simulink model "evtol_vehicle"  (R2024a)
settings: Solver=ode4  StartTime=0.0  StopTime=inf  FixedStep=0.01  RelTol=1e-3
values from neighbouring files (symbols this model uses):
  init_ned_m = waypoints(1:3,init_wypt_num)    [export_evtol_vehicle_fmu.m]
  init_rpy_rad = [0; waypoints(5,init_wypt_num); waypoints(4,init_wypt_num)] *pi/180    [export_evtol_vehicle_fmu.m]
  init_wypt_num = 1    [export_evtol_vehicle_fmu.m]
  max_hover_speed_mps = 15    [export_evtol_vehicle_fmu.m]
  num_waypoints = length(waypoints)    [export_evtol_vehicle_fmu.m]
  vdown_slew_rate_mps = 7.5    [export_evtol_vehicle_fmu.m]
  vx_slew_rate_mps = 7.5    [export_evtol_vehicle_fmu.m]
  vy_slew_rate_mps = 7.5    [export_evtol_vehicle_fmu.m]
  waypoints = [0 0 0 0 0 0 0 0 0 0 0 0 ... (900 elements, 9x100)]    [waypoints_empty.mat]
libraries: simulink x3, aerolibtransform2 x1
settings Model: Creator=cma  LastModifiedBy=Leo.Wong
settings OptimizationCC: ReuseModelBlockBuffer=off
settings RTWCC: GPUComputeCapability=3.5

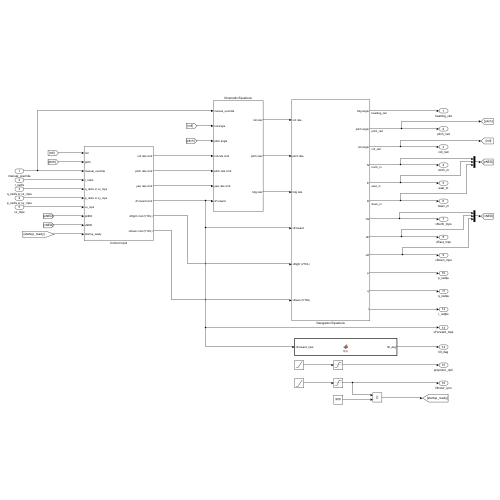
[thumbnail: Simulink's stored preview of the top-level diagram]
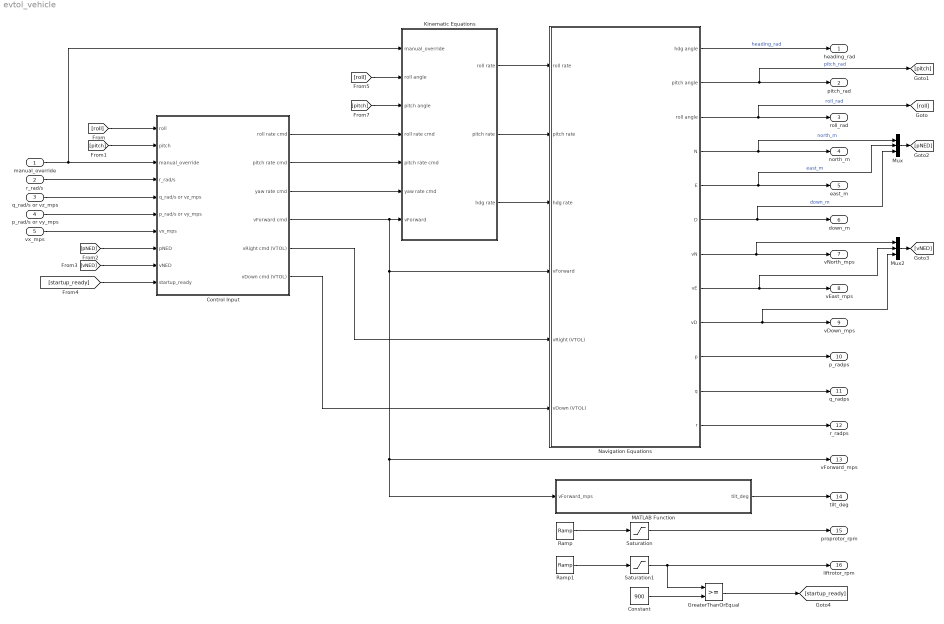
== system evtol_vehicle ==
  manual_override : Inport
  r_rad/s : Inport  Port=2
  q_rad/s or vz_mps : Inport  Port=3
  p_rad/s or vy_mps : Inport  Port=4
  vx_mps : Inport  Port=5
  Constant : Constant  Value=900
  Control Input : Subsystem  mask{wp_nedhgv=waypoints, num_wp=num_waypoints, initNED=init_ned_m, max_hover_speed=max_hover_speed_mps, vx_slew_rate=vx_slew_rate_mps, vy_slew_rate=vy_slew_rate_mps, vD_slew_rate=vdown_slew_rate_mps}
      mask prompts: wp_nedhgv "Waypoints"; num_wp "Number of Waypoints"; initNED "Initial NED (m)"; max_hover_speed "Max Hover Speed (mps)"; vx_slew_rate "Vx Slew Rate (mps)"; vy_slew_rate "Vy Slew Rate (mps)"; vD_slew_rate "VDown Slew Rate (mps)"
  GreaterThanOrEqual : RelationalOperator  OutDataTypeStr=boolean  RndMeth=Simplest  InputSameDT=off
  Kinematic Equations : Subsystem
  MATLAB Function : MATLAB Function  TreatAsAtomicUnit=on
  Mux : Mux  Inputs=3
  Mux2 : Mux  Inputs=3
  Navigation Equations : Subsystem  mask{initNED=init_ned_m, initRPY=init_rpy_rad}
      mask prompts: initNED "Initial NED (m)"; initRPY "Initial RPY (rad)"
  Ramp : simulink/Sources/Ramp  slope=600/5  start=0  InitialOutput=0
  Ramp1 : simulink/Sources/Ramp  slope=900/5  start=0  InitialOutput=0
  Saturation : Saturate  UpperLimit=600  LowerLimit=0
  Saturation1 : Saturate  UpperLimit=900  LowerLimit=0
  heading_rad : Outport
  pitch_rad : Outport  Port=2
  roll_rad : Outport  Port=3
  north_m : Outport  Port=4
  east_m : Outport  Port=5
  down_m : Outport  Port=6
  vNorth_mps : Outport  Port=7
  vEast_mps : Outport  Port=8
  vDown_mps : Outport  Port=9
  p_radps : Outport  Port=10
  q_radps : Outport  Port=11
  r_radps : Outport  Port=12
  vForward_mps : Outport  Port=13
  tilt_deg : Outport  Port=14
  proprotor_rpm : Outport  Port=15
  liftrotor_rpm : Outport  Port=16
  wires:
  Control Input/1(roll rate cmd) -> Kinematic Equations/4(roll rate cmd)
  Control Input/2(pitch rate cmd) -> Kinematic Equations/5(pitch rate cmd)
  Control Input/3(yaw rate cmd) -> Kinematic Equations/6(yaw rate cmd)
  [roll] -> Control Input/1(roll)
  [pitch] -> Control Input/2(pitch)
  Control Input/4(vForward cmd) -> Navigation Equations/4(vForward), MATLAB Function/1(vForward_mps), vForward_mps/1, Kinematic Equations/7(vForward)
  Control Input/6(vDown cmd (VTOL)) -> Navigation Equations/6(vDown (VTOL))
  Kinematic Equations/2(pitch rate) -> Navigation Equations/2(pitch rate)
  Kinematic Equations/1(roll rate) -> Navigation Equations/1(roll rate)
  Kinematic Equations/3(hdg rate) -> Navigation Equations/3(hdg rate)
  [roll] -> Kinematic Equations/2(roll angle)
  [pitch] -> Kinematic Equations/3(pitch angle)
  Control Input/5(vRight cmd (VTOL)) -> Navigation Equations/5(vRight (VTOL))
  r_rad/s/1 -> Control Input/4(r_rad/s)
  q_rad/s or vz_mps/1 -> Control Input/5(q_rad/s or vz_mps)
  p_rad/s or vy_mps/1 -> Control Input/6(p_rad/s or vy_mps)
  vx_mps/1 -> Control Input/7(vx_mps)
  Navigation Equations/4(N) -> Mux/1, north_m/1  "north_m"
  Navigation Equations/5(E) -> Mux/2, east_m/1  "east_m"
  Navigation Equations/6(D) -> Mux/3, down_m/1  "down_m"
  Navigation Equations/7(vN) -> Mux2/1, vNorth_mps/1
  Navigation Equations/8(vE) -> Mux2/2, vEast_mps/1
  Navigation Equations/9(vD) -> vDown_mps/1, Mux2/3
  Navigation Equations/10(p) -> p_radps/1
  Navigation Equations/11(q) -> q_radps/1
  Navigation Equations/12(r) -> r_radps/1
  Navigation Equations/3(roll angle) -> [roll], roll_rad/1  "roll_rad"
  Navigation Equations/2(pitch angle) -> [pitch], pitch_rad/1  "pitch_rad"
  Navigation Equations/1(hdg angle) -> heading_rad/1  "heading_rad"
  Mux/1 -> [pNED]
  Mux2/1 -> [vNED]
  manual_override/1 -> Kinematic Equations/1(manual_override), Control Input/3(manual_override)
  MATLAB Function/1(tilt_deg) -> tilt_deg/1
  Ramp/1 -> Saturation/1
  Ramp1/1 -> Saturation1/1
  Saturation/1 -> proprotor_rpm/1
  Saturation1/1 -> GreaterThanOrEqual/1, liftrotor_rpm/1
  [pNED] -> Control Input/8(pNED)
  [vNED] -> Control Input/9(vNED)
  GreaterThanOrEqual/1 -> [startup_ready]
  Constant/1 -> GreaterThanOrEqual/2
  [startup_ready] -> Control Input/10(startup_ready)

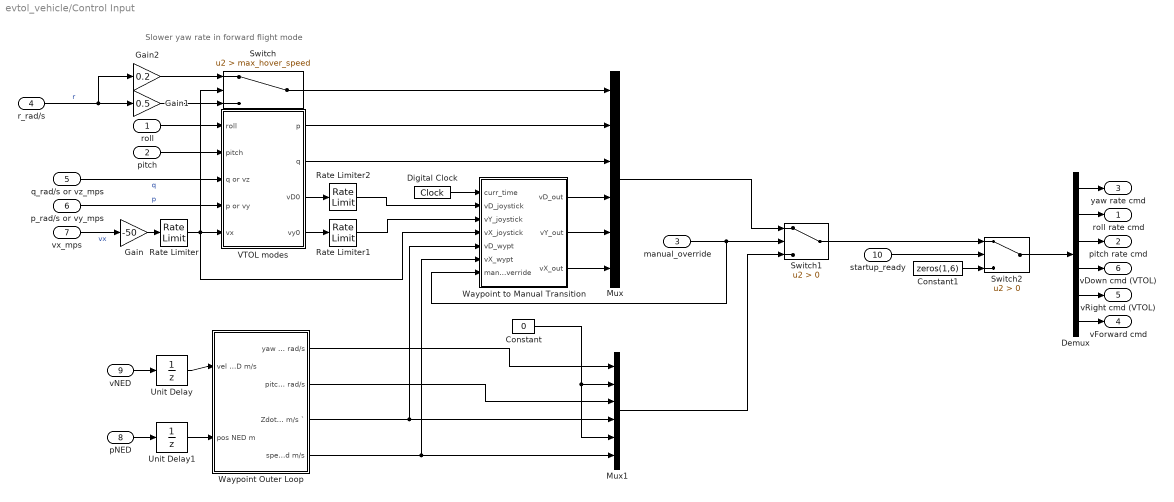
== system evtol_vehicle/Control Input ==
  note: Slower yaw rate in forward flight mode
  roll : Inport
  pitch : Inport  Port=2
  manual_override : Inport  Port=3
  r_rad/s : Inport  Port=4
  q_rad/s or vz_mps : Inport  Port=5
  p_rad/s or vy_mps : Inport  Port=6
  vx_mps : Inport  Port=7
  pNED : Inport  Port=8
  vNED : Inport  Port=9
  startup_ready : Inport  Port=10
  Constant : Constant  Value=0
  Constant1 : Constant  Value=zeros(1,6)
  Demux : Demux  Outputs=6
  Digital Clock : DigitalClock  SampleTime=0.01
  Gain : Gain  Gain=-50
  Gain1 : Gain  Gain=0.5
  Gain2 : Gain  Gain=0.2
  Mux : Mux  Inputs=6
  Mux1 : Mux  Inputs=6
  Rate Limiter : RateLimiter  RisingSlewLimit=vx_slew_rate  FallingSlewLimit=-vx_slew_rate  SampleTimeMode=inherited
  Rate Limiter1 : RateLimiter  RisingSlewLimit=vD_slew_rate  FallingSlewLimit=-vD_slew_rate  SampleTimeMode=inherited
  Rate Limiter2 : RateLimiter  RisingSlewLimit=vy_slew_rate  FallingSlewLimit=-vy_slew_rate  SampleTimeMode=inherited
  Switch : Switch  Criteria=u2 > Threshold  Threshold=max_hover_speed  SaturateOnIntegerOverflow=off  InputSameDT=off
  Switch1 : Switch  Criteria=u2 > Threshold  SaturateOnIntegerOverflow=off  InputSameDT=off
  Switch2 : Switch  Criteria=u2 > Threshold  SaturateOnIntegerOverflow=off  InputSameDT=off
  Unit Delay : UnitDelay  SampleTime=-1  HasFrameUpgradeWarning=on
  Unit Delay1 : UnitDelay  InitialCondition=initNED  SampleTime=-1  HasFrameUpgradeWarning=on
  VTOL modes : Subsystem
  Waypoint Outer Loop : Subsystem
  Waypoint to Manual Transition : MATLAB Function  TreatAsAtomicUnit=on  SystemSampleTime=0.01
  roll rate cmd : Outport
  pitch rate cmd : Outport  Port=2
  yaw rate cmd : Outport  Port=3
  vForward cmd : Outport  Port=4
  vRight cmd (VTOL) : Outport  Port=5
  vDown cmd (VTOL) : Outport  Port=6
  wires:
  Gain/1 -> Rate Limiter/1
  VTOL modes/3(vD0) -> Rate Limiter2/1
  r_rad/s/1 -> Gain2/1, Gain1/1  "r"
  p_rad/s or vy_mps/1 -> VTOL modes/4(p or vy)  "p"
  q_rad/s or vz_mps/1 -> VTOL modes/3(q or vz)  "q"
  vx_mps/1 -> Gain/1  "vx"
  roll/1 -> VTOL modes/1(roll)
  pitch/1 -> VTOL modes/2(pitch)
  VTOL modes/4(vy0) -> Rate Limiter1/1
  Gain2/1 -> Switch/1
  Gain1/1 -> Switch/3
  Rate Limiter/1 -> Waypoint to Manual Transition/4(vX_joystick), Switch/2, VTOL modes/5(vx)
  VTOL modes/2(q) -> Mux/3
  VTOL modes/1(p) -> Mux/2
  Mux/1 -> Switch1/1
  Demux/1 -> yaw rate cmd/1
  Demux/2 -> roll rate cmd/1
  Demux/3 -> pitch rate cmd/1
  Demux/4 -> vDown cmd (VTOL)/1
  Demux/5 -> vRight cmd (VTOL)/1
  Demux/6 -> vForward cmd/1
  Waypoint Outer Loop/4(speedCmd m/s) -> Waypoint to Manual Transition/6(vX_wypt), Mux1/6
  Waypoint Outer Loop/1(yaw rate rad/s) -> Mux1/1
  Waypoint Outer Loop/2(pitch rate rad/s) -> Mux1/3
  Waypoint Outer Loop/3(ZdotCmd m/s `) -> Waypoint to Manual Transition/5(vD_wypt), Mux1/4
  Mux1/1 -> Switch1/3
  Constant/1 -> Mux1/5, Mux1/2
  pNED/1 -> Unit Delay1/1
  manual_override/1 -> Waypoint to Manual Transition/7(manual_override), Switch1/2
  vNED/1 -> Unit Delay/1
  Switch/1 -> Mux/1
  Unit Delay/1 -> Waypoint Outer Loop/1(vel NED m/s)
  Unit Delay1/1 -> Waypoint Outer Loop/2(pos NED m)
  Switch1/1 -> Switch2/1
  Switch2/1 -> Demux/1
  startup_ready/1 -> Switch2/2
  Constant1/1 -> Switch2/3
  Digital Clock/1 -> Waypoint to Manual Transition/1(curr_time)
  Waypoint to Manual Transition/1(vD_out) -> Mux/4
  Waypoint to Manual Transition/2(vY_out) -> Mux/5
  Waypoint to Manual Transition/3(vX_out) -> Mux/6
  Rate Limiter2/1 -> Waypoint to Manual Transition/2(vD_joystick)
  Rate Limiter1/1 -> Waypoint to Manual Transition/3(vY_joystick)

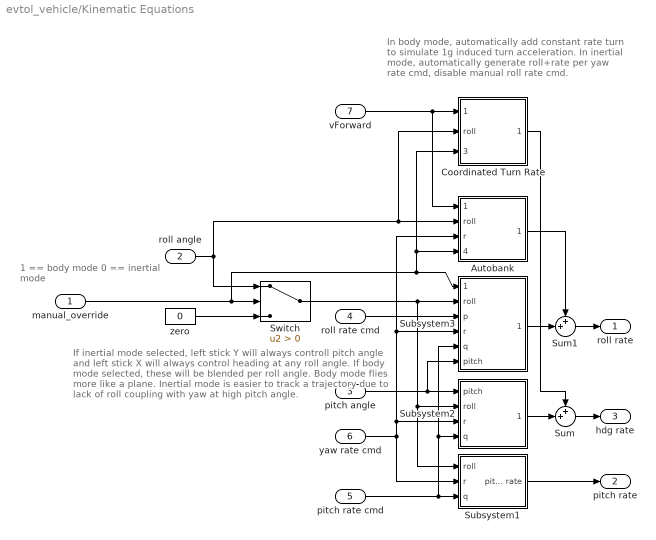
== system evtol_vehicle/Kinematic Equations ==
  note: If inertial mode selected, left stick Y will always controll pitch angle
      | and left stick X will always control heading at any roll angle.
      | If body mode selected, these will be blended per roll angle.
      | Body mode flies more like a plane.
      | Inertial mode is easier to track a trajectory due to lack
      | of roll coupling with yaw at high pitch angle.
  note: In body mode, automatically add constant rate
      | turn to simulate 1g induced turn acceleration.
      | In inertial mode, automatically generate roll+rate
      | per yaw rate cmd, disable manual roll rate cmd.
  note: 1 == body mode
      | 0 == inertial mode
  manual_override : Inport
  roll angle : Inport  Port=2
  pitch angle : Inport  Port=3
  roll rate cmd : Inport  Port=4
  pitch rate cmd : Inport  Port=5
  yaw rate cmd : Inport  Port=6
  vForward : Inport  Port=7
  Autobank : Subsystem
  Coordinated Turn Rate : Subsystem
  Subsystem1 : Subsystem
  Subsystem2 : Subsystem
  Subsystem3 : Subsystem
  Sum : Sum  Inputs=++|
  Sum1 : Sum  Inputs=++|
  Switch : Switch  Criteria=u2 > Threshold  SaturateOnIntegerOverflow=off  InputSameDT=off
  zero : Constant  Value=0
  roll rate : Outport
  pitch rate : Outport  Port=2
  hdg rate : Outport  Port=3
  wires:
  Subsystem1/1(pitch rate) -> pitch rate/1
  pitch rate cmd/1 -> Subsystem3/5(q), Subsystem2/4(q), Subsystem1/3(q)
  roll rate cmd/1 -> Subsystem3/3(p)
  yaw rate cmd/1 -> Subsystem1/2(r), Autobank/3(r), Subsystem3/4(r), Subsystem2/3(r)
  pitch angle/1 -> Subsystem3/6(pitch), Subsystem2/1(pitch)
  Switch/1 -> Subsystem1/1(roll), Subsystem2/2(roll), Subsystem3/2(roll)
  manual_override/1 -> Autobank/4(body mode), Coordinated Turn Rate/3(body mode), Subsystem3/1(body mode), Switch/2
  roll angle/1 -> Coordinated Turn Rate/2(roll), Autobank/2(roll), Switch/1
  zero/1 -> Switch/3
  Subsystem2/1(hdg rate) -> Sum/2
  Sum/1 -> hdg rate/1
  Coordinated Turn Rate/1(hdg rate) -> Sum/1
  vForward/1 -> Autobank/1(vForward), Coordinated Turn Rate/1(vForward)
  Sum1/1 -> roll rate/1
  Subsystem3/1(roll rate) -> Sum1/2
  Autobank/1(roll rate) -> Sum1/1

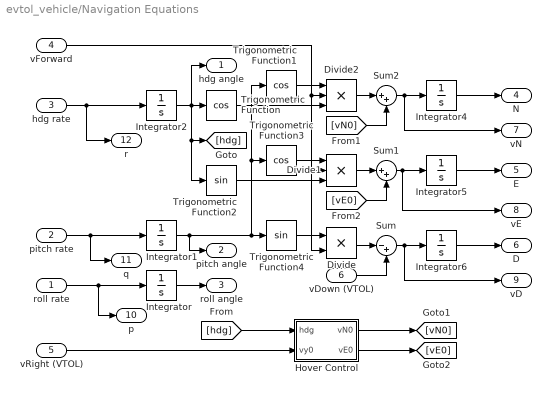
== system evtol_vehicle/Navigation Equations ==
  roll rate : Inport
  pitch rate : Inport  Port=2
  hdg rate : Inport  Port=3
  vForward : Inport  Port=4
  vRight (VTOL) : Inport  Port=5
  vDown (VTOL) : Inport  Port=6
  Divide : Product  Inputs=**
  Divide1 : Product  Inputs=***
  Divide2 : Product  Inputs=***
  Hover Control : Subsystem
  Integrator : Integrator  InitialCondition=initRPY(1)
  Integrator1 : Integrator  InitialCondition=initRPY(2)
  Integrator2 : Integrator  InitialCondition=initRPY(3)
  Integrator4 : Integrator  InitialCondition=initNED(1)
  Integrator5 : Integrator  InitialCondition=initNED(2)
  Integrator6 : Integrator  InitialCondition=initNED(3)
  Sum : Sum  Inputs=|-+
  Sum1 : Sum  Inputs=|++
  Sum2 : Sum  Inputs=|++
  Trigonometric Function : Trigonometry  Operator=cos
  Trigonometric Function1 : Trigonometry  Operator=cos
  Trigonometric Function2 : Trigonometry
  Trigonometric Function3 : Trigonometry  Operator=cos
  Trigonometric Function4 : Trigonometry
  hdg angle : Outport
  pitch angle : Outport  Port=2
  roll angle : Outport  Port=3
  N : Outport  Port=4
  E : Outport  Port=5
  D : Outport  Port=6
  vN : Outport  Port=7
  vE : Outport  Port=8
  vD : Outport  Port=9
  p : Outport  Port=10
  q : Outport  Port=11
  r : Outport  Port=12
  wires:
  Trigonometric Function3/1 -> Divide1/1
  Divide2/1 -> Sum2/1
  Trigonometric Function1/1 -> Divide2/1
  Sum/1 -> vD/1, Integrator6/1
  Divide/1 -> Sum/1
  Integrator1/1 -> pitch angle/1, Trigonometric Function1/1, Trigonometric Function3/1, Trigonometric Function4/1
  Divide1/1 -> Sum1/1
  Integrator2/1 -> hdg angle/1, [hdg], Trigonometric Function2/1, Trigonometric Function/1
  Trigonometric Function/1 -> Divide2/3
  Trigonometric Function4/1 -> Divide/1
  Sum2/1 -> vN/1, Integrator4/1
  Sum1/1 -> vE/1, Integrator5/1
  Trigonometric Function2/1 -> Divide1/3
  Integrator6/1 -> D/1
  vDown (VTOL)/1 -> Sum/2
  [vE0] -> Sum1/2
  [vN0] -> Sum2/2
  Integrator5/1 -> E/1
  Integrator4/1 -> N/1
  hdg rate/1 -> r/1, Integrator2/1
  roll rate/1 -> p/1, Integrator/1
  pitch rate/1 -> q/1, Integrator1/1
  Integrator/1 -> roll angle/1
  Hover Control/1(vN0) -> [vN0]
  Hover Control/2(vE0) -> [vE0]
  [hdg] -> Hover Control/1(hdg)
  vForward/1 -> Divide/2, Divide1/2, Divide2/2
  vRight (VTOL)/1 -> Hover Control/2(vy0)

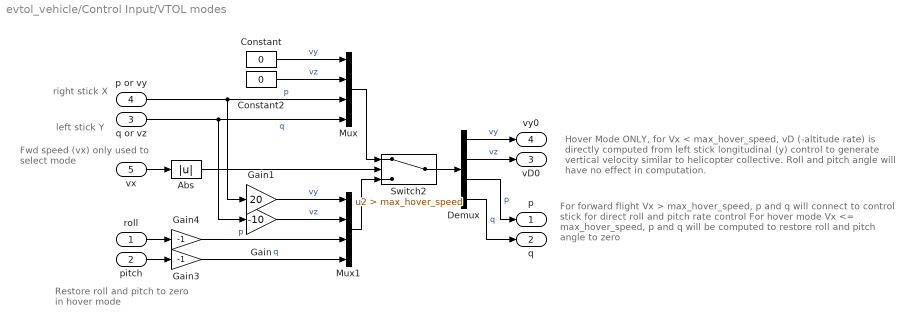
== system evtol_vehicle/Control Input/VTOL modes ==
  note: right stick X
  note: Fwd speed (vx) only
      | used to select mode
  note: Restore roll and pitch
      | to zero in hover mode
  note: Hover Mode ONLY, for Vx < max_hover_speed,
      | vD (-altitude rate) is directly computed from left stick longitudinal (y)
      | control to generate vertical velocity similar to helicopter collective.
      | Roll and pitch angle will have no effect in computation.
  note: For forward flight Vx > max_hover_speed, p and q will connect to
      | control stick for direct roll and pitch rate control
      |
      | For hover mode Vx <= max_hover_speed, p and q will be computed
      | to restore roll and pitch angle to zero
  note: left stick Y
  roll : Inport
  pitch : Inport  Port=2
  q or vz : Inport  Port=3
  p or vy : Inport  Port=4
  vx : Inport  Port=5
  Abs : Abs  SaturateOnIntegerOverflow=off
  Constant : Constant  Value=0
  Constant2 : Constant  Value=0
  Demux : Demux
  Gain : Gain  Gain=-10
  Gain1 : Gain  Gain=20
  Gain3 : Gain  Gain=-1
  Gain4 : Gain  Gain=-1
  Mux : Mux
  Mux1 : Mux
  Switch2 : Switch  Criteria=u2 > Threshold  Threshold=max_hover_speed  SaturateOnIntegerOverflow=off  InputSameDT=off
  p : Outport
  q : Outport  Port=2
  vD0 : Outport  Port=3
  vy0 : Outport  Port=4
  wires:
  Abs/1 -> Switch2/2
  Constant/1 -> Mux/1  "vy"
  vx/1 -> Abs/1
  p or vy/1 -> Gain1/1, Mux/3  "p"
  q or vz/1 -> Gain/1, Mux/4  "q"
  pitch/1 -> Gain3/1
  roll/1 -> Gain4/1
  Switch2/1 -> Demux/1
  Mux/1 -> Switch2/1
  Mux1/1 -> Switch2/3
  Gain1/1 -> Mux1/1  "vy"
  Constant2/1 -> Mux/2  "vz"
  Gain/1 -> Mux1/2  "vz"
  Gain3/1 -> Mux1/4  "q"
  Gain4/1 -> Mux1/3  "p"
  Demux/4 -> q/1  "q"
  Demux/3 -> p/1  "p"
  Demux/2 -> vD0/1  "vz"
  Demux/1 -> vy0/1  "vy"

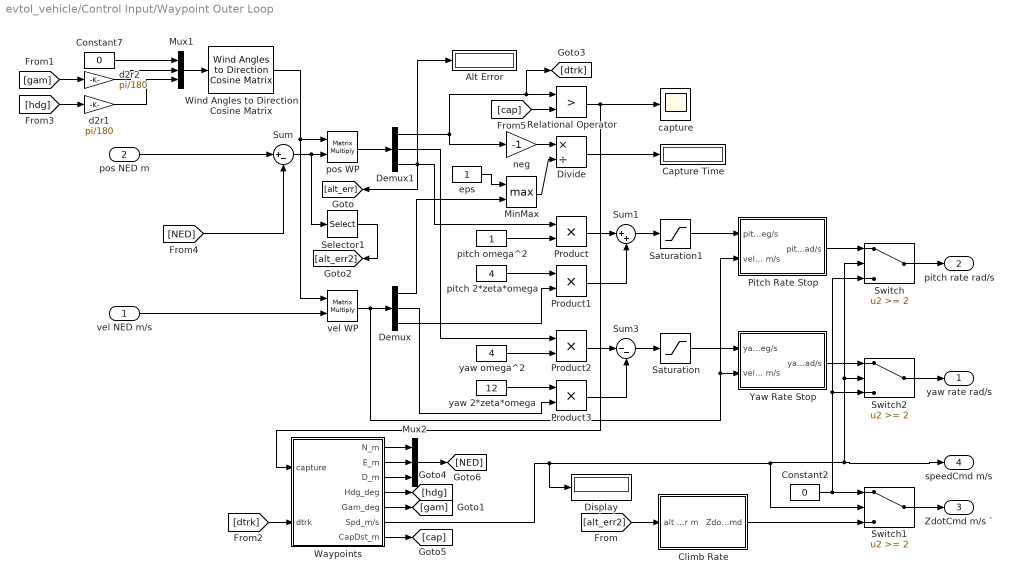
== system evtol_vehicle/Control Input/Waypoint Outer Loop ==
  vel NED m/s : Inport
  pos NED m : Inport  Port=2
  Alt Error : Display
  Capture Time : Display
  Climb Rate : Subsystem
  Constant2 : Constant  Value=0
  Constant7 : Constant  Value=0
  Demux : Demux  Outputs=3
  Demux1 : Demux  Outputs=3
  Display : Display
  Divide : Product  Inputs=*/
  MinMax : MinMax  Function=max  Inputs=2
  Mux1 : Mux  Inputs=3
  Mux2 : Mux  Inputs=3
  Pitch Rate Stop : Subsystem
  Product{,1..3} (4 alike) : Product
  Relational Operator : RelationalOperator  Operator=>  OutDataTypeStr=boolean  RndMeth=Simplest  InputSameDT=off
  Saturation : Saturate  UpperLimit=15  LowerLimit=-15
  Saturation1 : Saturate  UpperLimit=10  LowerLimit=-10
  Selector1 : Selector  InputPortWidth=3  IndexOptions=Index vector (dialog)  Indices=[3]  OutputSizes=1
  Sum : Sum  Inputs=|+-
  Sum1 : Sum  Inputs=|++
  Sum3 : Sum  Inputs=|--
  Switch : Switch  Threshold=2  SaturateOnIntegerOverflow=off  InputSameDT=off
  Switch1 : Switch  Threshold=2  SaturateOnIntegerOverflow=off  InputSameDT=off
  Switch2 : Switch  Threshold=2  SaturateOnIntegerOverflow=off  InputSameDT=off
  Waypoints : Subsystem
  Wind Angles to Direction Cosine Matrix : aerolibtransform2/Wind Angles to  Direction Cosine Matrix
  Yaw Rate Stop : Subsystem
  capture : Scope
  d2r1 : Gain  Gain=pi/180
  d2r2 : Gain  Gain=pi/180
  eps : Constant
  neg : Gain  Gain=-1
  pitch 2*zeta*omega : Constant  Value=4
  pitch omega^2 : Constant
  pos WP : Product  Multiplication=Matrix(*)
  vel WP : Product  Multiplication=Matrix(*)
  yaw 2*zeta*omega : Constant  Value=12
  yaw omega^2 : Constant  Value=4
  yaw rate rad/s : Outport
  pitch rate rad/s : Outport  Port=2
  ZdotCmd m/s ` : Outport  Port=3
  speedCmd m/s : Outport  Port=4
  wires:
  Sum/1 -> Selector1/1, pos WP/2
  Mux1/1 -> Wind Angles to Direction Cosine Matrix/1
  Constant7/1 -> Mux1/1
  Wind Angles to Direction Cosine Matrix/1 -> vel WP/1, pos WP/1
  pos WP/1 -> Demux1/1
  vel NED m/s/1 -> vel WP/2
  [NED] -> Sum/2
  pos NED m/1 -> Sum/1
  Demux1/1 -> neg/1, [dtrk], Relational Operator/1
  [cap] -> Relational Operator/2
  Relational Operator/1 -> capture/1, Waypoints/1(capture)
  Sum1/1 -> Saturation1/1
  Product/1 -> Sum1/1
  Product1/1 -> Sum1/2
  pitch omega^2/1 -> Product/2
  pitch 2*zeta*omega/1 -> Product1/1
  Demux1/3 -> [alt_err], Alt Error/1, Product/1
  yaw 2*zeta*omega/1 -> Product3/1
  yaw omega^2/1 -> Product2/2
  Product3/1 -> Sum3/2
  Product2/1 -> Sum3/1
  Sum3/1 -> Saturation/1
  Demux1/2 -> Product2/1
  neg/1 -> Divide/1
  Divide/1 -> Capture Time/1
  Demux/3 -> Product1/2
  Demux/2 -> Product3/2
  MinMax/1 -> Divide/2
  eps/1 -> MinMax/1
  Demux/1 -> MinMax/2
  vel WP/1 -> Pitch Rate Stop/2(vel WP m/s), Yaw Rate Stop/2(vel WP m/s), Demux/1
  Saturation1/1 -> Pitch Rate Stop/1(pitch rate Cmd deg/s)
  Waypoints/6(Spd_m/s) -> Display/1, Switch/2, Switch2/2, speedCmd m/s/1, Switch1/2
  d2r1/1 -> Mux1/3
  d2r2/1 -> Mux1/2
  Pitch Rate Stop/1(pitch rate rad/s) -> Switch/1
  Switch/1 -> pitch rate rad/s/1
  Constant2/1 -> Switch1/1, Switch2/3, Switch/3
  [alt_err2] -> Climb Rate/1(alt error m)
  Switch1/1 -> ZdotCmd m/s `/1
  Climb Rate/1(ZdotCmd) -> Switch1/3
  Saturation/1 -> Yaw Rate Stop/1(yaw rate Cmd deg/s)
  Selector1/1 -> [alt_err2]
  [dtrk] -> Waypoints/2(dtrk)
  Waypoints/5(Gam_deg) -> [gam]
  Waypoints/4(Hdg_deg) -> [hdg]
  Waypoints/7(CapDst_m) -> [cap]
  [hdg] -> d2r1/1
  [gam] -> d2r2/1
  Waypoints/1(N_m) -> Mux2/1
  Waypoints/2(E_m) -> Mux2/2
  Waypoints/3(D_m) -> Mux2/3
  Mux2/1 -> [NED]
  Yaw Rate Stop/1(yaw rate rad/s) -> Switch2/1
  Switch2/1 -> yaw rate rad/s/1

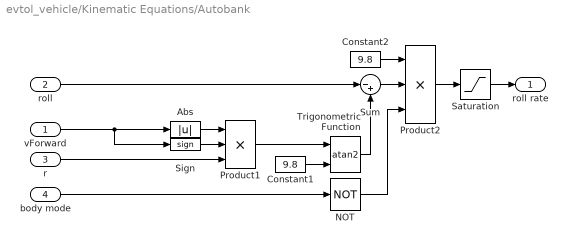
== system evtol_vehicle/Kinematic Equations/Autobank ==
  vForward : Inport
  roll : Inport  Port=2
  r : Inport  Port=3
  body mode : Inport  Port=4
  Abs : Abs  SaturateOnIntegerOverflow=off
  Constant1 : Constant  Value=9.8
  Constant2 : Constant  Value=9.8
  NOT : Logic  Operator=NOT  IconShape=distinctive  AllPortsSameDT=off  OutDataTypeStr=boolean
  Product1 : Product  Inputs=3
  Product2 : Product  Inputs=3
  Saturation : Saturate  UpperLimit=45*pi/180  LowerLimit=-45*pi/180
  Sign : Signum
  Sum : Sum  Inputs=|-+
  Trigonometric Function : Trigonometry  Operator=atan2
  roll rate : Outport
  wires:
  Abs/1 -> Product1/1
  Product1/1 -> Trigonometric Function/1
  vForward/1 -> Sign/1, Abs/1
  Constant1/1 -> Trigonometric Function/2
  roll/1 -> Sum/1
  Trigonometric Function/1 -> Sum/2
  Product2/1 -> Saturation/1
  Sum/1 -> Product2/2
  Constant2/1 -> Product2/1
  body mode/1 -> NOT/1
  NOT/1 -> Product2/3
  Sign/1 -> Product1/2
  r/1 -> Product1/3
  Saturation/1 -> roll rate/1

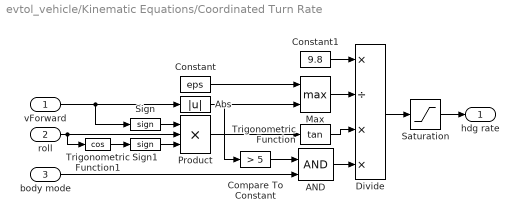
== system evtol_vehicle/Kinematic Equations/Coordinated Turn Rate ==
  vForward : Inport
  roll : Inport  Port=2
  body mode : Inport  Port=3
  AND : Logic  IconShape=distinctive  AllPortsSameDT=off  OutDataTypeStr=boolean
  Abs : Abs  SaturateOnIntegerOverflow=off
  Compare To Constant : simulink/Logic and Bit Operations/Compare To Constant  relop=>  const=5  OutDataTypeStr=boolean
  Constant : Constant  Value=eps
  Constant1 : Constant  Value=9.8
  Divide : Product  Inputs=*/**
  Max : MinMax  Function=max  Inputs=2
  Product : Product  Inputs=3
  Saturation : Saturate  UpperLimit=1  LowerLimit=-1
  Sign : Signum
  Sign1 : Signum
  Trigonometric Function : Trigonometry  Operator=tan
  Trigonometric Function1 : Trigonometry  Operator=cos
  hdg rate : Outport
  wires:
  Sign/1 -> Product/1
  Constant/1 -> Max/1
  Constant1/1 -> Divide/1
  vForward/1 -> Sign/1, Abs/1
  Product/1 -> Trigonometric Function/1
  Divide/1 -> Saturation/1
  Max/1 -> Divide/2
  Compare To Constant/1 -> AND/1
  AND/1 -> Divide/4
  Saturation/1 -> hdg rate/1
  Trigonometric Function/1 -> Divide/3
  Abs/1 -> Compare To Constant/1, Max/2
  body mode/1 -> AND/2
  roll/1 -> Product/2, Trigonometric Function1/1
  Sign1/1 -> Product/3
  Trigonometric Function1/1 -> Sign1/1

== system evtol_vehicle/Kinematic Equations/Subsystem1 ==
  roll : Inport
  r : Inport  Port=2
  q : Inport  Port=3
  Divide4 : Product  Inputs=**
  Divide6 : Product  Inputs=**
  Sum : Sum  Inputs=|+-
  Trigonometric Function7 : Trigonometry  Operator=cos
  Trigonometric Function8 : Trigonometry
  pitch rate : Outport
  wires:
  r/1 -> Divide6/2
  Trigonometric Function8/1 -> Divide6/1
  Divide6/1 -> Sum/2
  Trigonometric Function7/1 -> Divide4/2
  Divide4/1 -> Sum/1
  Sum/1 -> pitch rate/1
  roll/1 -> Trigonometric Function7/1, Trigonometric Function8/1
  q/1 -> Divide4/1

== system evtol_vehicle/Kinematic Equations/Subsystem2 ==
  pitch : Inport
  roll : Inport  Port=2
  r : Inport  Port=3
  q : Inport  Port=4
  Divide : Product  Inputs=*/
  Divide3 : Product  Inputs=**
  Divide5 : Product  Inputs=**
  Sum1 : Sum  Inputs=++|
  Trigonometric Function1 : Trigonometry  Operator=cos
  Trigonometric Function5 : Trigonometry  Operator=cos
  Trigonometric Function6 : Trigonometry
  hdg rate : Outport
  wires:
  roll/1 -> Trigonometric Function5/1, Trigonometric Function6/1
  Trigonometric Function5/1 -> Divide3/2
  r/1 -> Divide3/1
  Trigonometric Function6/1 -> Divide5/1
  Divide5/1 -> Sum1/2
  Divide3/1 -> Sum1/1
  q/1 -> Divide5/2
  pitch/1 -> Trigonometric Function1/1
  Sum1/1 -> Divide/1
  Divide/1 -> hdg rate/1
  Trigonometric Function1/1 -> Divide/2

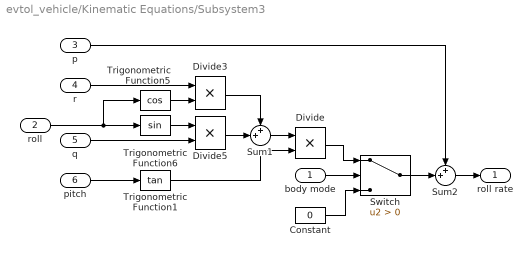
== system evtol_vehicle/Kinematic Equations/Subsystem3 ==
  body mode : Inport
  roll : Inport  Port=2
  p : Inport  Port=3
  r : Inport  Port=4
  q : Inport  Port=5
  pitch : Inport  Port=6
  Constant : Constant  Value=0
  Divide : Product  Inputs=**
  Divide3 : Product  Inputs=**
  Divide5 : Product  Inputs=**
  Sum1 : Sum  Inputs=++|
  Sum2 : Sum  Inputs=++|
  Switch : Switch  Criteria=u2 > Threshold  SaturateOnIntegerOverflow=off  InputSameDT=off
  Trigonometric Function1 : Trigonometry  Operator=tan
  Trigonometric Function5 : Trigonometry  Operator=cos
  Trigonometric Function6 : Trigonometry
  roll rate : Outport
  wires:
  Trigonometric Function1/1 -> Divide/2
  Sum1/1 -> Divide/1
  pitch/1 -> Trigonometric Function1/1
  q/1 -> Divide5/2
  Trigonometric Function6/1 -> Divide5/1
  r/1 -> Divide3/1
  Trigonometric Function5/1 -> Divide3/2
  roll/1 -> Trigonometric Function6/1, Trigonometric Function5/1
  Divide5/1 -> Sum1/2
  Divide3/1 -> Sum1/1
  Sum2/1 -> roll rate/1
  p/1 -> Sum2/1
  body mode/1 -> Switch/2
  Divide/1 -> Switch/1
  Switch/1 -> Sum2/2
  Constant/1 -> Switch/3

== system evtol_vehicle/Navigation Equations/Hover Control ==
  note: heading is used to distribute
      | lateral velocity vy to vN and vE
  note: Hover Mode ONLY, for Vx < max_hover_speed_mps,
      | vE and vN are directly computed from right stick lateral (x)
      | control to generate lateral translation velocity based on heading.
      | Roll and pitch angle will have no effect in compuation.
  hdg : Inport
  vy0 : Inport  Port=2
  Constant1 : Constant  Value=-1
  Product : Product  Inputs=3
  Product1 : Product
  Trigonometric Function : Trigonometry  Operator=cos
  Trigonometric Function1 : Trigonometry
  vN0 : Outport
  vE0 : Outport  Port=2
  wires:
  vy0/1 -> Product1/2, Product/2
  Product1/1 -> vE0/1
  Trigonometric Function1/1 -> Product/1
  Product/1 -> vN0/1
  hdg/1 -> Trigonometric Function1/1, Trigonometric Function/1
  Constant1/1 -> Product/3
  Trigonometric Function/1 -> Product1/1

== system evtol_vehicle/Control Input/Waypoint Outer Loop/Climb Rate ==
  alt error m : Inport
  Constant3 : Constant  Value=-1
  Product5 : Product
  Saturation2 : Saturate  UpperLimit=5  LowerLimit=-5
  ZdotCmd : Outport
  wires:
  Constant3/1 -> Product5/2
  Product5/1 -> Saturation2/1
  alt error m/1 -> Product5/1
  Saturation2/1 -> ZdotCmd/1

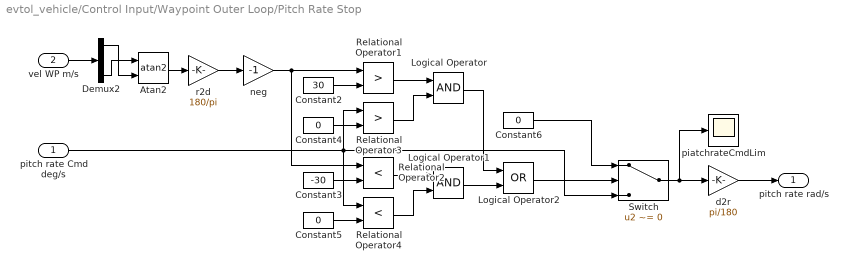
== system evtol_vehicle/Control Input/Waypoint Outer Loop/Pitch Rate Stop ==
  pitch rate Cmd deg/s : Inport
  vel WP m/s : Inport  Port=2
  Atan2 : Trigonometry  Operator=atan2
  Constant2 : Constant  Value=30
  Constant3 : Constant  Value=-30
  Constant4 : Constant  Value=0
  Constant5 : Constant  Value=0
  Constant6 : Constant  Value=0
  Demux2 : Demux  Outputs=3
  Logical Operator : Logic  AllPortsSameDT=off  OutDataTypeStr=boolean
  Logical Operator1 : Logic  AllPortsSameDT=off  OutDataTypeStr=boolean
  Logical Operator2 : Logic  Operator=OR  AllPortsSameDT=off  OutDataTypeStr=boolean
  Relational Operator1 : RelationalOperator  Operator=>  OutDataTypeStr=boolean  RndMeth=Simplest  InputSameDT=off
  Relational Operator2 : RelationalOperator  Operator=<  OutDataTypeStr=boolean  RndMeth=Simplest  InputSameDT=off
  Relational Operator3 : RelationalOperator  Operator=>  OutDataTypeStr=boolean  RndMeth=Simplest  InputSameDT=off
  Relational Operator4 : RelationalOperator  Operator=<  OutDataTypeStr=boolean  RndMeth=Simplest  InputSameDT=off
  Switch : Switch  Criteria=u2 ~= 0  SaturateOnIntegerOverflow=off  InputSameDT=off
  d2r : Gain  Gain=pi/180
  neg : Gain  Gain=-1
  piatchrateCmdLim : Scope
  r2d : Gain  Gain=180/pi
  pitch rate rad/s : Outport
  wires:
  vel WP m/s/1 -> Demux2/1
  Demux2/1 -> Atan2/2
  Atan2/1 -> r2d/1
  d2r/1 -> pitch rate rad/s/1
  Constant4/1 -> Relational Operator3/2
  Logical Operator/1 -> Logical Operator2/1
  Constant2/1 -> Relational Operator1/2
  neg/1 -> Relational Operator1/1, Relational Operator2/1
  Relational Operator3/1 -> Logical Operator/2
  Relational Operator1/1 -> Logical Operator/1
  Logical Operator2/1 -> Switch/2
  Relational Operator2/1 -> Logical Operator1/1
  Constant3/1 -> Relational Operator2/2
  Constant6/1 -> Switch/1
  Relational Operator4/1 -> Logical Operator1/2
  Logical Operator1/1 -> Logical Operator2/2
  Constant5/1 -> Relational Operator4/2
  Switch/1 -> piatchrateCmdLim/1, d2r/1
  Demux2/3 -> Atan2/1
  pitch rate Cmd deg/s/1 -> Relational Operator4/1, Switch/3, Relational Operator3/1
  r2d/1 -> neg/1

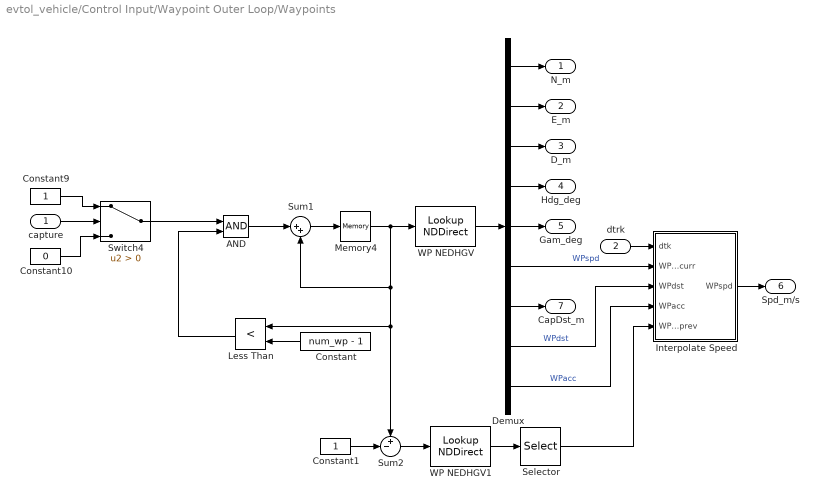
== system evtol_vehicle/Control Input/Waypoint Outer Loop/Waypoints ==
  capture : Inport
  dtrk : Inport  Port=2
  AND : Logic  IconShape=distinctive  AllPortsSameDT=off  OutDataTypeStr=boolean
  Constant : Constant  Value=num_wp - 1
  Constant1 : Constant
  Constant10 : Constant  Value=0
  Constant9 : Constant
  Demux : Demux  Outputs=9
  Interpolate Speed : Subsystem
  Less Than : RelationalOperator  Operator=<  OutDataTypeStr=boolean  RndMeth=Simplest  InputSameDT=off
  Memory4 : Memory  InitialCondition=init_wypt_num
  Selector : Selector  InputPortWidth=9  IndexOptions=Index vector (dialog)  Indices=[6]  OutputSizes=1
  Sum1 : Sum  Inputs=|++
  Sum2 : Sum  Inputs=+-|
  Switch4 : Switch  Criteria=u2 > Threshold  SaturateOnIntegerOverflow=off  InputSameDT=off
  WP NEDHGV : LookupNDDirect  InputsSelectThisObjectFromTable=Vector  Table=wp_nedhgv
  WP NEDHGV1 : LookupNDDirect  InputsSelectThisObjectFromTable=Vector  Table=wp_nedhgv
  N_m : Outport
  E_m : Outport  Port=2
  D_m : Outport  Port=3
  Hdg_deg : Outport  Port=4
  Gam_deg : Outport  Port=5
  Spd_m/s : Outport  Port=6
  CapDst_m : Outport  Port=7
  wires:
  capture/1 -> Switch4/2
  Constant9/1 -> Switch4/1
  Constant10/1 -> Switch4/3
  Switch4/1 -> AND/1
  Memory4/1 -> Sum1/2, Sum2/1, Less Than/1, WP NEDHGV/1
  Sum1/1 -> Memory4/1
  Demux/5 -> Gam_deg/1
  Demux/4 -> Hdg_deg/1
  Demux/1 -> N_m/1
  Demux/2 -> E_m/1
  Demux/6 -> Interpolate Speed/2(WPspd_curr)  "WPspd"
  Demux/3 -> D_m/1
  WP NEDHGV/1 -> Demux/1
  WP NEDHGV1/1 -> Selector/1
  Sum2/1 -> WP NEDHGV1/1
  Constant1/1 -> Sum2/2
  Demux/7 -> CapDst_m/1
  dtrk/1 -> Interpolate Speed/1(dtk)
  Selector/1 -> Interpolate Speed/5(WPspd_prev)
  Demux/9 -> Interpolate Speed/4(WPacc)  "WPacc"
  Demux/8 -> Interpolate Speed/3(WPdst)  "WPdst"
  Interpolate Speed/1(WPspd) -> Spd_m/s/1
  Constant/1 -> Less Than/2
  Less Than/1 -> AND/2
  AND/1 -> Sum1/1

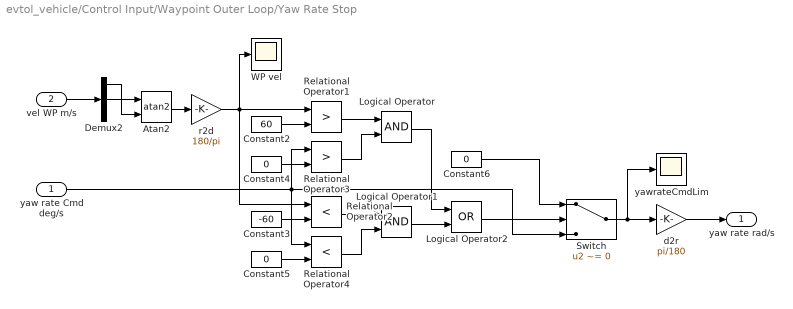
== system evtol_vehicle/Control Input/Waypoint Outer Loop/Yaw Rate Stop ==
  yaw rate Cmd deg/s : Inport
  vel WP m/s : Inport  Port=2
  Atan2 : Trigonometry  Operator=atan2
  Constant2 : Constant  Value=60
  Constant3 : Constant  Value=-60
  Constant4 : Constant  Value=0
  Constant5 : Constant  Value=0
  Constant6 : Constant  Value=0
  Demux2 : Demux  Outputs=3
  Logical Operator : Logic  AllPortsSameDT=off  OutDataTypeStr=boolean
  Logical Operator1 : Logic  AllPortsSameDT=off  OutDataTypeStr=boolean
  Logical Operator2 : Logic  Operator=OR  AllPortsSameDT=off  OutDataTypeStr=boolean
  Relational Operator1 : RelationalOperator  Operator=>  OutDataTypeStr=boolean  RndMeth=Simplest  InputSameDT=off
  Relational Operator2 : RelationalOperator  Operator=<  OutDataTypeStr=boolean  RndMeth=Simplest  InputSameDT=off
  Relational Operator3 : RelationalOperator  Operator=>  OutDataTypeStr=boolean  RndMeth=Simplest  InputSameDT=off
  Relational Operator4 : RelationalOperator  Operator=<  OutDataTypeStr=boolean  RndMeth=Simplest  InputSameDT=off
  Switch : Switch  Criteria=u2 ~= 0  SaturateOnIntegerOverflow=off  InputSameDT=off
  WP vel : Scope
  d2r : Gain  Gain=pi/180
  r2d : Gain  Gain=180/pi
  yawrateCmdLim : Scope
  yaw rate rad/s : Outport
  wires:
  Switch/1 -> d2r/1, yawrateCmdLim/1
  Constant5/1 -> Relational Operator4/2
  Logical Operator1/1 -> Logical Operator2/2
  Relational Operator4/1 -> Logical Operator1/2
  yaw rate Cmd deg/s/1 -> Relational Operator3/1, Switch/3, Relational Operator4/1
  Constant6/1 -> Switch/1
  Constant3/1 -> Relational Operator2/2
  Relational Operator2/1 -> Logical Operator1/1
  Logical Operator2/1 -> Switch/2
  Relational Operator1/1 -> Logical Operator/1
  Relational Operator3/1 -> Logical Operator/2
  r2d/1 -> WP vel/1, Relational Operator2/1, Relational Operator1/1
  Constant2/1 -> Relational Operator1/2
  Logical Operator/1 -> Logical Operator2/1
  Constant4/1 -> Relational Operator3/2
  d2r/1 -> yaw rate rad/s/1
  Atan2/1 -> r2d/1
  Demux2/1 -> Atan2/2
  Demux2/2 -> Atan2/1
  vel WP m/s/1 -> Demux2/1

== system evtol_vehicle/Control Input/Waypoint Outer Loop/Waypoints/Interpolate Speed ==
  dtk : Inport
  WPspd_curr : Inport  Port=2
  WPdst : Inport  Port=3
  WPacc : Inport  Port=4
  WPspd_prev : Inport  Port=5
  Divide : Product  Inputs=/*
  Product : Product
  Saturation : Saturate  UpperLimit=1  LowerLimit=0
  Sum2 : Sum  Inputs=|+-
  Sum3 : Sum  Inputs=|++
  Sum4 : Sum  Inputs=|++
  WPspd : Outport
  wires:
  WPspd_prev/1 -> Sum2/2, Sum3/2
  Product/1 -> Sum3/1
  Saturation/1 -> Product/2
  dtk/1 -> Sum4/1
  Divide/1 -> Saturation/1
  Sum2/1 -> Product/1
  WPdst/1 -> Sum4/2
  WPspd_curr/1 -> Sum2/1
  Sum3/1 -> WPspd/1
  Sum4/1 -> Divide/2
  WPacc/1 -> Divide/1

== matlab function evtol_vehicle/Control Input/Waypoint to Manual Transition ==
  data: curr_time input; vD_joystick input; vY_joystick input; vX_joystick input; vD_out output; vD_wypt input; vX_wypt input; manual_override input; vY_out output; vX_out output
function [vD_out, vY_out, vX_out] = fcn(curr_time, vD_joystick, vY_joystick, vX_joystick, vD_wypt, vX_wypt, manual_override)

persistent start_time;
persistent dD;
persistent dY;
persistent dX;
transition_duration_s = 2.0;

if(manual_override && isempty(start_time))
    dD = vD_wypt - vD_joystick;
    dX = vX_wypt - vX_joystick;
    dY = -vY_joystick;
    start_time = curr_time;
end

if(~isempty(start_time) && curr_time - start_time < transition_duration_s)
    elapsed_time_s = curr_time - start_time;
    vD_out = (dD*(transition_duration_s-elapsed_time_s)/transition_duration_s) + vD_joystick;
    vX_out = (dX*(transition_duration_s-elapsed_time_s)/transition_duration_s) + vX_joystick;
    vY_out = (dY*(transition_duration_s-elapsed_time_s)/transition_duration_s) + vY_joystick;

else
    vD_out = vD_joystick;
    vX_out = vX_joystick;
    vY_out = vY_joystick;
end

== matlab function evtol_vehicle/MATLAB Function ==
  data: vForward_mps input; tilt_deg output
function tilt_deg = fcn(vForward_mps)

if vForward_mps < 0
    tilt_deg = 0.0;
    return;
end

tilt_deg = min(1.0, vForward_mps/25.0) * 90.0;
